simulink model "solar_panel_power_test"  (R2016b)
settings: Solver=VariableStepAuto  StartTime=0.0  StopTime=500  RelTol=1e-3
values from neighbouring files (symbols this model uses):
  fsw_params = init_fsw_params()    [init_solar_panel_power_test.m]
libraries: GPS_time_lib x1, aerolibtransform2 x1, dynamics_lib x1, solar_panel_power_lib x1, sun_vector_lib x1, target_generation_lib x1, time_coord_rotation_lib x1, tle2eci_coarse_lib x1
settings Model: Creator=taylorreynolds  LastModifiedBy=taylorreynolds

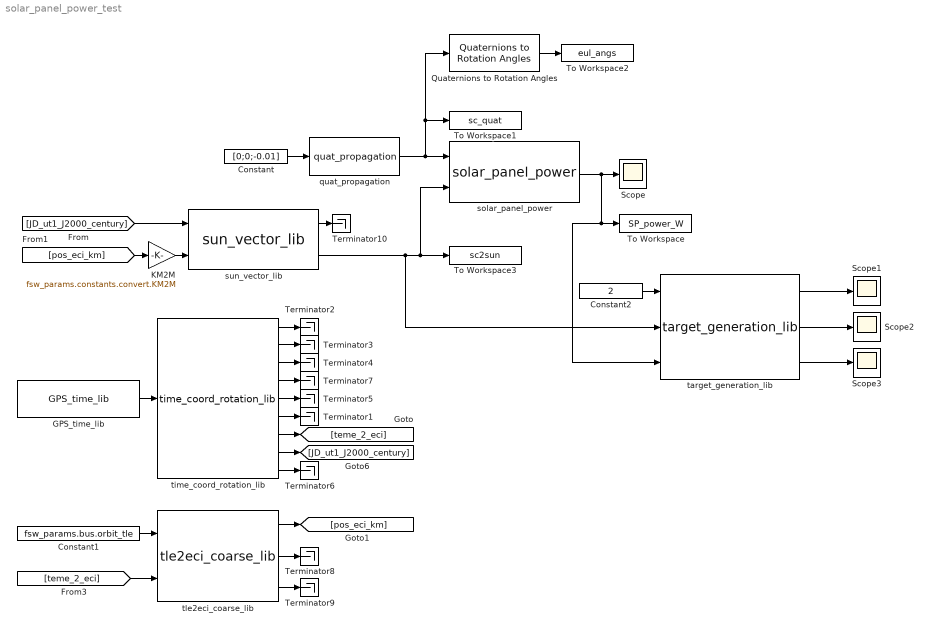
== system solar_panel_power_test ==
  Constant : Constant  Value=[0;0;-0.01]
  Constant1 : Constant  Value=fsw_params.bus.orbit_tle
  Constant2 : Constant  Value=2  OutDataTypeStr=int8
  GPS_time_lib : GPS_time_lib/GPS_time_lib
  KM2M : Gain  Gain=fsw_params.constants.convert.KM2M
  Quaternions to Rotation Angles : aerolibtransform2/Quaternions to Rotation Angles  rotationOrder=XYZ
  Scope{,1..3} (4 alike) : Scope
  Terminator{1..10} (10 alike) : Terminator
  To Workspace : ToWorkspace  VariableName=SP_power_W  SaveFormat=Structure With Time  SampleTime=-1
  To Workspace1 : ToWorkspace  VariableName=sc_quat  SaveFormat=Structure With Time  SampleTime=-1
  To Workspace2 : ToWorkspace  VariableName=eul_angs  SaveFormat=Structure With Time  SampleTime=-1
  To Workspace3 : ToWorkspace  VariableName=sc2sun  SaveFormat=Structure With Time  SampleTime=-1
  quat_propagation : dynamics_lib/Dynamics/quat_propagation
  solar_panel_power : solar_panel_power_lib/solar_panel_power
  sun_vector_lib : sun_vector_lib/sun_vector_lib
  target_generation_lib : target_generation_lib/target_generation_lib
  time_coord_rotation_lib : time_coord_rotation_lib/time_coord_rotation_lib
  tle2eci_coarse_lib : tle2eci_coarse_lib/tle2eci_coarse_lib
  wires:
  quat_propagation/1 -> Quaternions to Rotation Angles/1, To Workspace1/1, solar_panel_power/1
  Constant1/1 -> tle2eci_coarse_lib/1
  GPS_time_lib/1 -> time_coord_rotation_lib/1
  time_coord_rotation_lib/2 -> Terminator3/1
  time_coord_rotation_lib/3 -> Terminator4/1
  time_coord_rotation_lib/4 -> Terminator7/1
  time_coord_rotation_lib/5 -> Terminator5/1
  time_coord_rotation_lib/8 -> [JD_ut1_J2000_century]
  time_coord_rotation_lib/7 -> [teme_2_eci]
  time_coord_rotation_lib/6 -> Terminator1/1
  time_coord_rotation_lib/1 -> Terminator2/1
  [JD_ut1_J2000_century] -> sun_vector_lib/1
  time_coord_rotation_lib/9 -> Terminator6/1
  [teme_2_eci] -> tle2eci_coarse_lib/2
  sun_vector_lib/2 -> target_generation_lib/2, To Workspace3/1, solar_panel_power/2
  tle2eci_coarse_lib/1 -> [pos_eci_km]
  tle2eci_coarse_lib/2 -> Terminator8/1
  tle2eci_coarse_lib/3 -> Terminator9/1
  sun_vector_lib/1 -> Terminator10/1
  KM2M/1 -> sun_vector_lib/2
  [pos_eci_km] -> KM2M/1
  Constant/1 -> quat_propagation/1
  solar_panel_power/1 -> target_generation_lib/3, To Workspace/1, Scope/1
  Quaternions to Rotation Angles/1 -> To Workspace2/1
  Constant2/1 -> target_generation_lib/1
  target_generation_lib/2 -> Scope2/1
  target_generation_lib/3 -> Scope3/1
  target_generation_lib/1 -> Scope1/1
